simulink model "RAM_test"  (R2019a)
settings: Solver=VariableStepAuto  StartTime=0.0  StopTime=stop_time  RelTol=1e-3
InitFcn:
  | sm_callback_init
undefined symbols (not defined in the file): a, b, B_k_0_init, c, calib_bpfs, F_bits, FIR_0_Size, FIR_0_Uprate, mp, Ts, W_bits
libraries: simulink x13, dsphdlfiltering x1, hdlsllib x1
settings Model: Creator=Balad  LastModifiedBy=Bailey

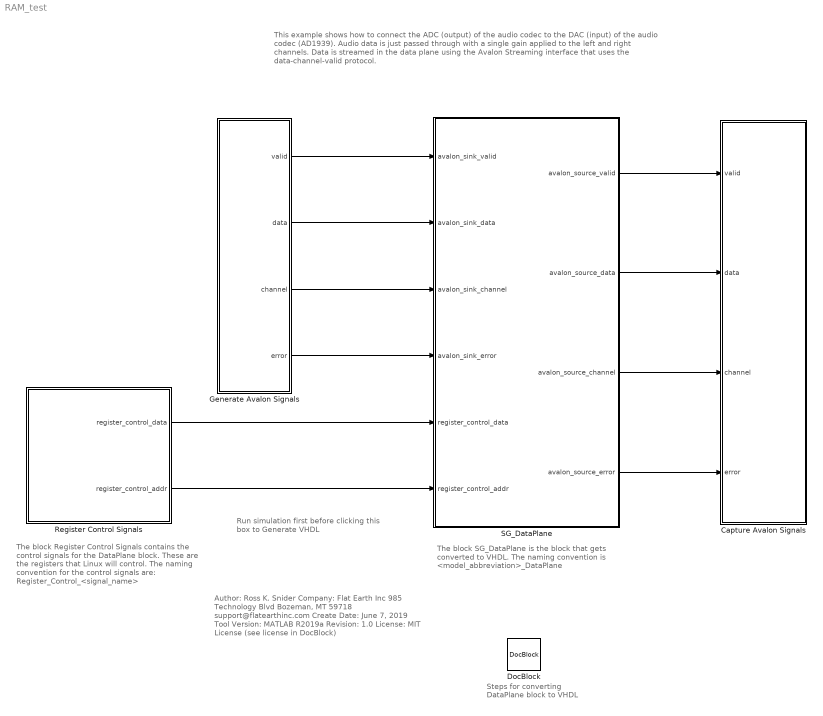
== system RAM_test ==
  note: Author:          Ross K. Snider
      | Company:     Flat Earth Inc
      |                       985 Technology Blvd
      |                       Bozeman, MT 59718
      |                       support@flatearthinc.com
      | Create Date:  June 7, 2019
      | Tool Version:  MATLAB R2019a
      | Revision:        1.0
      | License:          MIT License (see license in DocBlock)
  note: The block SG_DataPlane is the block that gets
      | converted to VHDL. The naming convention is
      | <model_abbreviation>_DataPlane
  note: Steps for converting
      | DataPlane block
      | to VHDL
  note: This example shows how to connect the ADC (output) of the audio codec to the DAC (input) of the audio codec (AD1939). Audio data is just passed through with a single gain applied to the left and right channels. Data is streamed in the data plane using the Avalon Streaming interface that uses the data-channel-valid protocol.
  note: The block Register Control Signals contains
      | the control signals for the DataPlane block.
      | These are the registers that Linux will control.
      | The naming convention for the control
      | signals are:  Register_Control_<signal_name>
  note: Run simulation first
      | before clicking this box to
      | Generate VHDL
  Capture Avalon Signals : Subsystem
  DocBlock : simulink/Model-Wide Utilities/DocBlock  DocumentType=HTML
      content=|
      | <html><head></head><body>
      | Type your documentation here</body></html>
  Generate Avalon Signals : Subsystem
  Register Control Signals : Subsystem
  SG_DataPlane : Subsystem  TreatAsAtomicUnit=on
  wires:
  Register Control Signals/2(register_control_addr) -> SG_DataPlane/6(register_control_addr)
  SG_DataPlane/2(avalon_source_data) -> Capture Avalon Signals/2(data)
  Generate Avalon Signals/3(channel) -> SG_DataPlane/3(avalon_sink_channel)
  Register Control Signals/1(register_control_data) -> SG_DataPlane/5(register_control_data)
  Generate Avalon Signals/2(data) -> SG_DataPlane/2(avalon_sink_data)
  Generate Avalon Signals/1(valid) -> SG_DataPlane/1(avalon_sink_valid)
  SG_DataPlane/4(avalon_source_error) -> Capture Avalon Signals/4(error)
  Generate Avalon Signals/4(error) -> SG_DataPlane/4(avalon_sink_error)
  SG_DataPlane/3(avalon_source_channel) -> Capture Avalon Signals/3(channel)
  SG_DataPlane/1(avalon_source_valid) -> Capture Avalon Signals/1(valid)

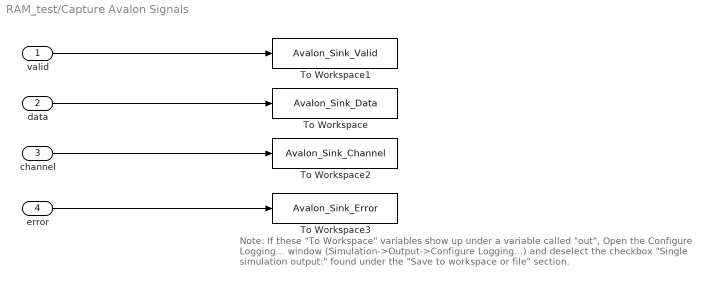
== system RAM_test/Capture Avalon Signals ==
  note: Note:  If these "To Workspace" variables show up under a variable called "out",
      | Open the Configure Logging... window (Simulation->Output->Configure Logging...)
      | and deselect the checkbox "Single simulation output:" found under the "Save to workspace or file" section.
  valid : Inport
  data : Inport  Port=2
  channel : Inport  Port=3
  error : Inport  Port=4
  To Workspace : ToWorkspace  VariableName=Avalon_Sink_Data  SaveFormat=Timeseries  SampleTime=-1
  To Workspace1 : ToWorkspace  VariableName=Avalon_Sink_Valid  SaveFormat=Timeseries  SampleTime=-1
  To Workspace2 : ToWorkspace  VariableName=Avalon_Sink_Channel  SaveFormat=Timeseries  SampleTime=-1
  To Workspace3 : ToWorkspace  VariableName=Avalon_Sink_Error  SaveFormat=Timeseries  SampleTime=-1
  wires:
  data/1 -> To Workspace/1
  valid/1 -> To Workspace1/1
  error/1 -> To Workspace3/1
  channel/1 -> To Workspace2/1

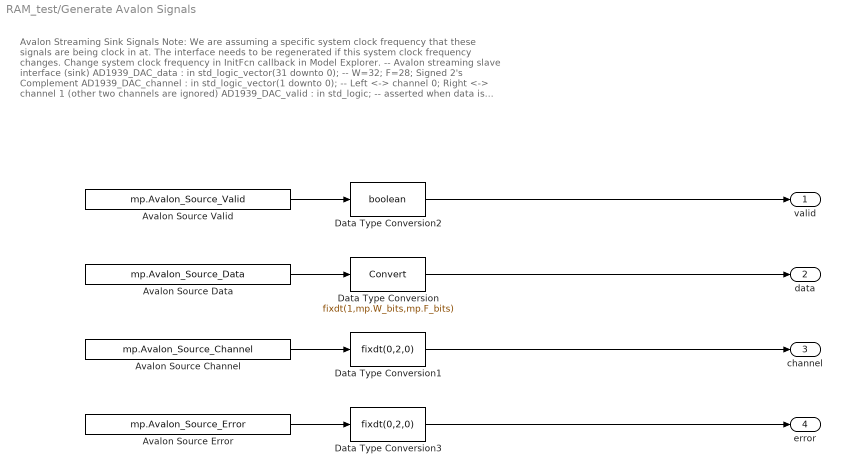
== system RAM_test/Generate Avalon Signals ==
  note: Avalon Streaming Sink Signals
      | Note: We are assuming a specific system clock frequency that these signals are being clock in at.
      | The interface needs to be regenerated if this system clock frequency changes. Change system clock frequency in InitFcn callback in Model Explorer.
      |
      | -- Avalon streaming slave interface (sink)
      | AD1939_DAC_data : in std_logic_vector(31 downto 0); -- W=32; F=28; Signed 2's Complement
      | AD1939_DAC_channel : in std_logic_vector(1 downto 0); -- Left <-> channel 0; Right <-> channel 1 (other two channels are ignored)
      | AD1939_DAC_valid : in std_logic; -- asserted when data is valid
      | AD1939_DAC_error : in std_logic_vector(1 downto 0) -- error channel is ignored, assumed to be error free at this point
      |
      | For more information on the data-channel-valid protocol, see chapter 5 in Intel's Avalon Interfaced Specification (p. 40) at https://www.intel.com/content/dam/www/programmable/us/en/pdfs/literature/manual/mnl_avalon_spec.pdf
  Avalon Source Channel : FromWorkspace  VariableName=mp.Avalon_Source_Channel  OutDataTypeStr=double  SampleTime=mp.Ts_system
  "Avalon Source Data " : FromWorkspace  VariableName=mp.Avalon_Source_Data  OutDataTypeStr=double  SampleTime=mp.Ts_system
  Avalon Source Error : FromWorkspace  VariableName=mp.Avalon_Source_Error  OutDataTypeStr=double  SampleTime=mp.Ts_system
  Avalon Source Valid : FromWorkspace  VariableName=mp.Avalon_Source_Valid  OutDataTypeStr=double  SampleTime=mp.Ts_system
  Data Type Conversion : DataTypeConversion  OutDataTypeStr=fixdt(1,mp.W_bits,mp.F_bits)
  Data Type Conversion1 : DataTypeConversion  OutDataTypeStr=fixdt(0,2,0)
  Data Type Conversion2 : DataTypeConversion  OutDataTypeStr=boolean
  Data Type Conversion3 : DataTypeConversion  OutDataTypeStr=fixdt(0,2,0)
  valid : Outport
  data : Outport  Port=2
  channel : Outport  Port=3
  error : Outport  Port=4
  wires:
  Data Type Conversion1/1 -> channel/1
  Data Type Conversion2/1 -> valid/1
  Avalon Source Error/1 -> Data Type Conversion3/1
  Data Type Conversion/1 -> data/1
  Avalon Source Valid/1 -> Data Type Conversion2/1
  Data Type Conversion3/1 -> error/1
  Avalon Source Channel/1 -> Data Type Conversion1/1
  "Avalon Source Data "/1 -> Data Type Conversion/1

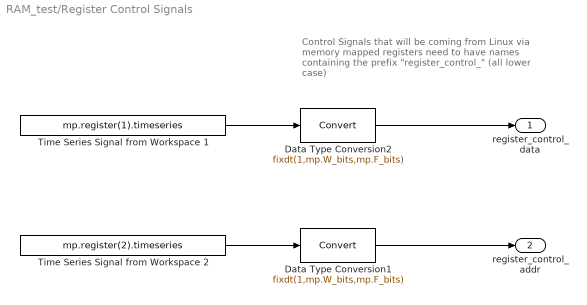
== system RAM_test/Register Control Signals ==
  note: Control Signals that will be coming from Linux via
      | memory mapped registers need to have names
      | containing the prefix "register_control_"
      | (all lower case)
  Data Type Conversion1 : DataTypeConversion  OutDataTypeStr=fixdt(1,mp.W_bits,mp.F_bits)
  Data Type Conversion2 : DataTypeConversion  OutDataTypeStr=fixdt(1,mp.W_bits,mp.F_bits)
  Time Series Signal from Workspace 1 : FromWorkspace  VariableName=mp.register(1).timeseries  OutDataTypeStr=double  SampleTime=mp.Ts_system
  Time Series Signal from Workspace 2 : FromWorkspace  VariableName=mp.register(2).timeseries  OutDataTypeStr=double  SampleTime=mp.Ts_system
  register_control_data : Outport
  register_control_addr : Outport  Port=2
  wires:
  Time Series Signal from Workspace 1/1 -> Data Type Conversion2/1
  Time Series Signal from Workspace 2/1 -> Data Type Conversion1/1
  Data Type Conversion2/1 -> register_control_data/1
  Data Type Conversion1/1 -> register_control_addr/1

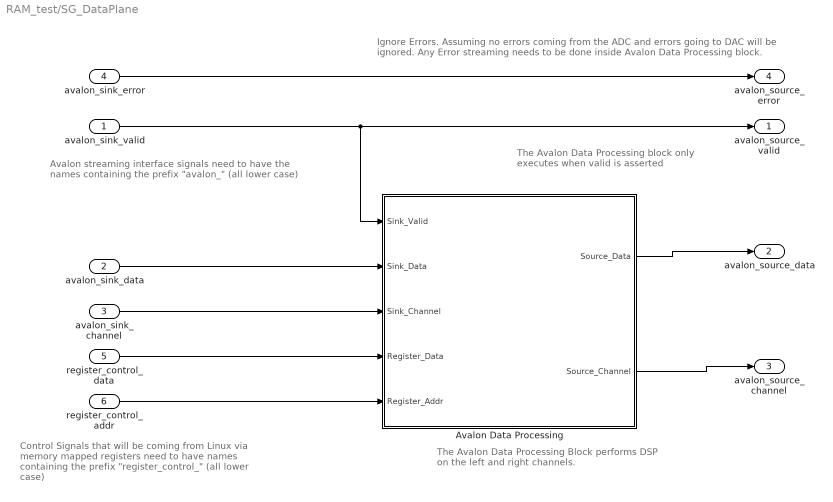
== system RAM_test/SG_DataPlane ==
  note: Control Signals that will be coming from Linux via
      | memory mapped registers need to have names
      | containing the prefix "register_control_"
      | (all lower case)
  note: The Avalon Data Processing Block
      | performs DSP on the left and right channels.
  note: The Avalon Data Processing block
      | only executes when valid is asserted
  note: Ignore Errors.
      | Assuming no errors coming from the ADC and errors going to DAC will be ignored.
      | Any Error streaming needs to be done inside Avalon Data Processing block.
  note: Avalon streaming interface signals need to have the
      | names containing the prefix "avalon_"
      | (all lower case)
  avalon_sink_valid : Inport
  avalon_sink_data : Inport  Port=2
  avalon_sink_channel : Inport  Port=3
  avalon_sink_error : Inport  Port=4
  register_control_data : Inport  Port=5
  register_control_addr : Inport  Port=6
  Avalon Data Processing : Subsystem  TreatAsAtomicUnit=on
  avalon_source_valid : Outport
  avalon_source_data : Outport  Port=2
  avalon_source_channel : Outport  Port=3
  avalon_source_error : Outport  Port=4
  wires:
  avalon_sink_channel/1 -> Avalon Data Processing/3(Sink_Channel)
  avalon_sink_error/1 -> avalon_source_error/1
  Avalon Data Processing/1(Source_Data) -> avalon_source_data/1
  avalon_sink_valid/1 -> avalon_source_valid/1, Avalon Data Processing/1(Sink_Valid)
  avalon_sink_data/1 -> Avalon Data Processing/2(Sink_Data)
  Avalon Data Processing/2(Source_Channel) -> avalon_source_channel/1
  register_control_addr/1 -> Avalon Data Processing/5(Register_Addr)
  register_control_data/1 -> Avalon Data Processing/4(Register_Data)

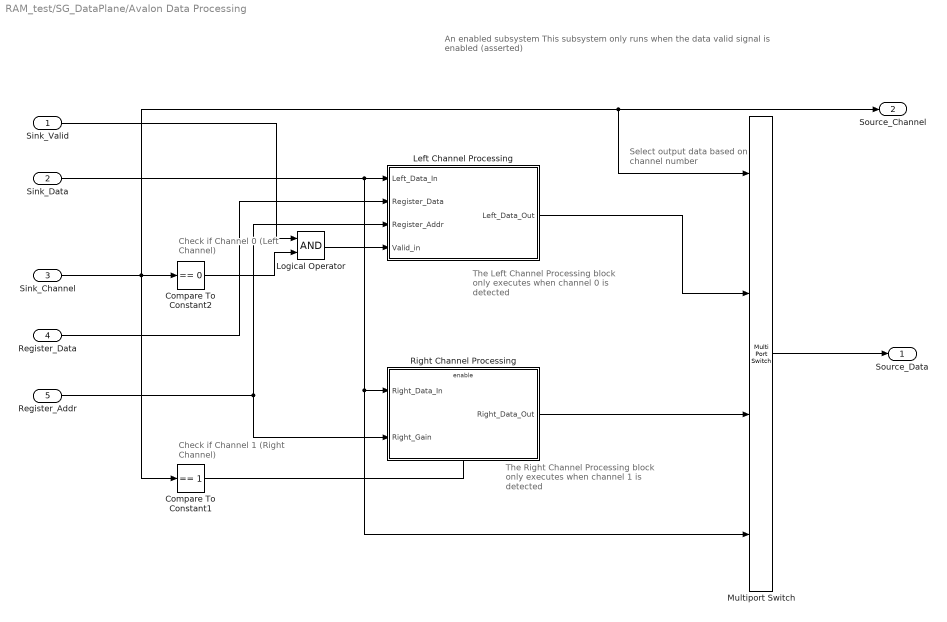
== system RAM_test/SG_DataPlane/Avalon Data Processing ==
  note: Select output data
      | based on channel number
  note: Check if Channel 0
      | (Left Channel)
  note: The Left Channel Processing block
      | only executes when channel 0
      | is detected
  note: The Right Channel Processing block
      | only executes when channel 1
      | is detected
  note: Check if Channel 1
      | (Right Channel)
  note: An enabled subsystem
      | This subsystem only runs when the data valid signal is enabled (asserted)
  Sink_Valid : Inport
  Sink_Data : Inport  Port=2
  Sink_Channel : Inport  Port=3
  Register_Data : Inport  Port=4
  Register_Addr : Inport  Port=5
  Compare To Constant1 : simulink/Logic and Bit Operations/Compare To Constant  relop===  const=1  OutDataTypeStr=boolean
  Compare To Constant2 : simulink/Logic and Bit Operations/Compare To Constant  relop===  const=0  OutDataTypeStr=boolean
  Left Channel Processing : Subsystem  TreatAsAtomicUnit=on
  Logical Operator : Logic  AllPortsSameDT=off  OutDataTypeStr=boolean
  Multiport Switch : MultiPortSwitch  DataPortOrder=Zero-based contiguous  DiagnosticForDefault=None  zeroidx=on
  Right Channel Processing : Subsystem  TreatAsAtomicUnit=on
  Source_Data : Outport  InitialOutput=0
  Source_Channel : Outport  Port=2  InitialOutput=0
  wires:
  Sink_Channel/1 -> Source_Channel/1, Multiport Switch/1, Compare To Constant1/1, Compare To Constant2/1
  Compare To Constant2/1 -> Logical Operator/2
  Compare To Constant1/1 -> Right Channel Processing/Enable
  Sink_Data/1 -> Multiport Switch/4, Right Channel Processing/1(Right_Data_In), Left Channel Processing/1(Left_Data_In)
  Left Channel Processing/1("Left_Data_Out ") -> Multiport Switch/2
  Right Channel Processing/1("Right_Data_Out ") -> Multiport Switch/3
  Multiport Switch/1 -> Source_Data/1
  Register_Data/1 -> Left Channel Processing/2(Register_Data)
  Register_Addr/1 -> Left Channel Processing/3(Register_Addr), Right Channel Processing/2(Right_Gain)
  Logical Operator/1 -> Left Channel Processing/4(Valid_in)
  Sink_Valid/1 -> Logical Operator/1

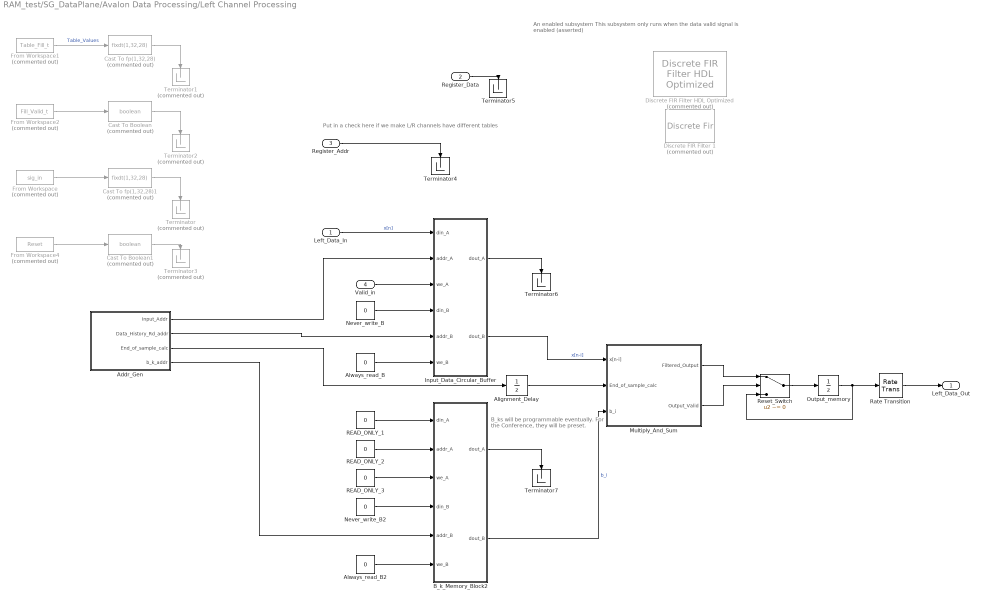
== system RAM_test/SG_DataPlane/Avalon Data Processing/Left Channel Processing ==
  note: B_ks will be programmable eventually.
      | For the Conference, they will be preset.
  note: Put in a check here if we make L/R channels have different tables
  note: An enabled subsystem
      | This subsystem only runs when the data valid signal is enabled (asserted)
  Left_Data_In : Inport
  Register_Data : Inport  Port=2
  Register_Addr : Inport  Port=3
  Valid_in : Inport  Port=4
  "Addr_Gen " : Subsystem
  Alignment_Delay : UnitDelay  SampleTime=-1  HasFrameUpgradeWarning=on
  Always_read_B : Constant  Value=0  OutDataTypeStr=boolean  SampleTime=Ts/FIR_0_Uprate
  Always_read_B2 : Constant  Value=0  OutDataTypeStr=boolean  SampleTime=Ts/FIR_0_Uprate
  B_k_Memory_Block2 : Subsystem  AncestorBlock=DualPortRam_UNLOCKED/Dual Rate Dual Port RAM1  mask(Dual-rate dual-port RAM){ram_size=FIR_0_Size}
      mask prompts: ram_size "Address port width (2 to 28 bits)"
      mask help: This block simulates a dual-clock dual-port RAM with two data output ports.
      mask init:
      | hdlblkmask_drdpram();
      mask Help: helpview([docroot '/simulink/helptargets.map'],'HDL_dual_rate_dual_port_ram');
  Cast To Boolean : DataTypeConversion  Commented=on  OutDataTypeStr=boolean
  Cast To Boolean1 : DataTypeConversion  Commented=on  OutDataTypeStr=boolean
  Cast To fp(1,32,28) : DataTypeConversion  Commented=on  OutDataTypeStr=fixdt(1,32,28)  RndMeth=Round
  Cast To fp(1,32,28)1 : DataTypeConversion  Commented=on  OutDataTypeStr=fixdt(1,32,28)  RndMeth=Round
  Discrete FIR Filter HDL Optimized : dsphdlfiltering/Discrete FIR Filter HDL Optimized  Commented=on  NumeratorSource=Property  Numerator=calib_bpfs(2:calib_bpfs(1,1)+1 ,1)'  NumeratorPrototype=[]  FilterStructure=Direct form systolic  SerializationOption=Minimum number of cycles between valid input samples  NumberOfCycles=2  NumberOfMultipliers=2  SimulateUsing=Code generation  roundingMode=Floor  overflowMode=off  CoefficientsDataTypeStr=fixdt(1, W_bits, F_bits)  CoefficientsMin=[]  CoefficientsMax=[]  OutputDataTypeStr=fixdt(1, W_bits, F_bits)  OutputMin=[]  OutputMax=[]  ResetInputPort=off  HDLGlobalReset=off
      settings: SourceProductName=DSP System Toolbox  SourceProductBaseCode=DS
  Discrete FIR Filter 1 : DiscreteFir  Commented=on  Coefficients=calib_bpfs(2:calib_bpfs(1,1)+1 ,1)'  CoefDataTypeStr=fixdt(1, W_bits, F_bits)  ProductDataTypeStr=fixdt(1, W_bits, F_bits)  AccumDataTypeStr=fixdt(1, W_bits, F_bits)  OutDataTypeStr=fixdt(1, W_bits, F_bits)
  From Workspace : FromWorkspace  Commented=on  VariableName=sig_in  SampleTime=Ts  OutputAfterFinalValue=Setting to zero
  From Workspace1 : FromWorkspace  Commented=on  VariableName=Table_Fill_t  SampleTime=Ts  Interpolate=off  OutputAfterFinalValue=Setting to zero
  From Workspace2 : FromWorkspace  Commented=on  VariableName=Fill_Valid_t  SampleTime=Ts  OutputAfterFinalValue=Setting to zero
  From Workspace4 : FromWorkspace  Commented=on  VariableName=Reset  SampleTime=Ts  Interpolate=off  OutputAfterFinalValue=Setting to zero
  Input_Data_Circular_Buffer : Subsystem  AncestorBlock=DualPortRam_UNLOCKED/Dual Rate Dual Port RAM1  mask(Dual-rate dual-port RAM){ram_size=FIR_0_Size}
      mask prompts: ram_size "Address port width (2 to 28 bits)"
      mask help: This block simulates a dual-clock dual-port RAM with two data output ports.
      mask init:
      | hdlblkmask_drdpram();
      mask Help: helpview([docroot '/simulink/helptargets.map'],'HDL_dual_rate_dual_port_ram');
  Multiply_And_Sum : Subsystem
  Never_write_B : Constant  Value=0  OutDataTypeStr=fixdt(1,W_bits, F_bits)  SampleTime=Ts/FIR_0_Uprate
  Never_write_B2 : Constant  Value=0  OutDataTypeStr=fixdt(1,W_bits, F_bits)  SampleTime=Ts/FIR_0_Uprate
  Output_memory : UnitDelay  SampleTime=-1  HasFrameUpgradeWarning=on
  READ_ONLY_1 : Constant  Value=0  OutDataTypeStr=fixdt(1,W_bits, F_bits)  SampleTime=Ts/FIR_0_Uprate
  READ_ONLY_2 : Constant  Value=0  OutDataTypeStr=fixdt(0,FIR_0_Size, 0)  SampleTime=Ts/FIR_0_Uprate
  READ_ONLY_3 : Constant  Value=0  OutDataTypeStr=boolean  SampleTime=Ts/FIR_0_Uprate
  Rate Transition : RateTransition  OutPortSampleTime=Ts
  Reset_Switch : Switch  Criteria=u2 ~= 0
  Terminator{,1..3} (4 alike) : Terminator  Commented=on
  Terminator{4..7} (4 alike) : Terminator
  "Left_Data_Out " : Outport  InitialOutput=0
  wires:
  Cast To Boolean1/1 -> Terminator3/1
  Cast To Boolean/1 -> Terminator2/1
  Cast To fp(1,32,28)1/1 -> Terminator/1
  From Workspace1/1 -> Cast To fp(1,32,28)/1  "Table_Values"
  Output_memory/1 -> Rate Transition/1, Reset_Switch/3
  From Workspace2/1 -> Cast To Boolean/1
  From Workspace/1 -> Cast To fp(1,32,28)1/1
  From Workspace4/1 -> Cast To Boolean1/1
  Cast To fp(1,32,28)/1 -> Terminator1/1
  Left_Data_In/1 -> Input_Data_Circular_Buffer/1(din_A)  "x[n]"
  Register_Data/1 -> Terminator5/1
  Register_Addr/1 -> Terminator4/1
  Valid_in/1 -> Input_Data_Circular_Buffer/3(we_A)
  Input_Data_Circular_Buffer/1(dout_A) -> Terminator6/1
  Never_write_B/1 -> Input_Data_Circular_Buffer/4(din_B)
  "Addr_Gen "/1(Input_Addr) -> Input_Data_Circular_Buffer/2(addr_A)
  "Addr_Gen "/2(Data_History_Rd_addr) -> Input_Data_Circular_Buffer/5(addr_B)
  Always_read_B/1 -> Input_Data_Circular_Buffer/6(we_B)
  Input_Data_Circular_Buffer/2(dout_B) -> Multiply_And_Sum/1(x[n-i])  "x[n-i]"
  READ_ONLY_1/1 -> B_k_Memory_Block2/1(din_A)
  READ_ONLY_3/1 -> B_k_Memory_Block2/3(we_A)
  READ_ONLY_2/1 -> B_k_Memory_Block2/2(addr_A)
  Never_write_B2/1 -> B_k_Memory_Block2/4(din_B)
  "Addr_Gen "/4(b_k_addr) -> B_k_Memory_Block2/5(addr_B)
  Always_read_B2/1 -> B_k_Memory_Block2/6(we_B)
  B_k_Memory_Block2/1(dout_A) -> Terminator7/1
  B_k_Memory_Block2/2(dout_B) -> Multiply_And_Sum/3(b_i)  "b_i"
  "Addr_Gen "/3(End_of_sample_calc) -> Alignment_Delay/1
  Reset_Switch/1 -> Output_memory/1
  Multiply_And_Sum/2(Output_Valid) -> Reset_Switch/2
  Multiply_And_Sum/1(Filtered_Output) -> Reset_Switch/1
  Rate Transition/1 -> "Left_Data_Out "/1
  Alignment_Delay/1 -> Multiply_And_Sum/2(End_of_sample_calc)

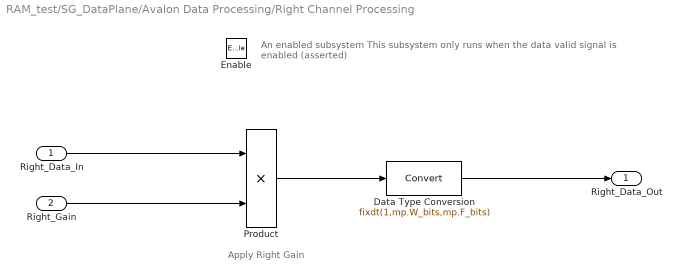
== system RAM_test/SG_DataPlane/Avalon Data Processing/Right Channel Processing ==
  note: Apply Right Gain
  note: An enabled subsystem
      | This subsystem only runs when the data valid signal is enabled (asserted)
  Right_Data_In : Inport
  Right_Gain : Inport  Port=2
  Enable : EnablePort
  Data Type Conversion : DataTypeConversion  OutDataTypeStr=fixdt(1,mp.W_bits,mp.F_bits)
  Product : Product
  "Right_Data_Out " : Outport  InitialOutput=0
  wires:
  Data Type Conversion/1 -> "Right_Data_Out "/1
  Product/1 -> Data Type Conversion/1
  Right_Data_In/1 -> Product/1
  Right_Gain/1 -> Product/2

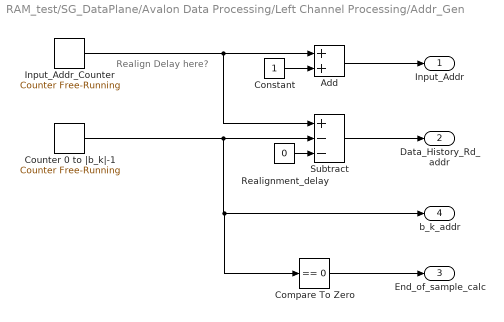
== system RAM_test/SG_DataPlane/Avalon Data Processing/Left Channel Processing/Addr_Gen  ==
  note: Realign Delay here?
  Add : Sum  OutDataTypeStr=Inherit: Same as first input
  Compare To Zero : simulink/Logic and Bit Operations/Compare To Zero  relop===  OutDataTypeStr=boolean  ZeroCross=off
  Constant : Constant  OutDataTypeStr=fixdt(0, FIR_0_Size,0)  SampleTime=-1
  Counter 0 to |b_k|-1 : simulink/Sources/Counter Free-Running  NumBits=FIR_0_Size  tsamp=Ts/FIR_0_Uprate
  Input_Addr_Counter : simulink/Sources/Counter Free-Running  NumBits=FIR_0_Size  tsamp=Ts
  Realignment_delay : Constant  Value=0  OutDataTypeStr=fixdt(0, FIR_0_Size,0)  SampleTime=-1
  Subtract : Sum  Inputs=+--  OutDataTypeStr=Inherit: Same as first input
  Input_Addr : Outport
  Data_History_Rd_addr : Outport  Port=2
  End_of_sample_calc : Outport  Port=3
  b_k_addr : Outport  Port=4
  wires:
  Counter 0 to |b_k|-1/1 -> Subtract/2, Compare To Zero/1, b_k_addr/1
  Subtract/1 -> Data_History_Rd_addr/1
  Input_Addr_Counter/1 -> Add/1, Subtract/1
  Add/1 -> Input_Addr/1
  Constant/1 -> Add/2
  Realignment_delay/1 -> Subtract/3
  Compare To Zero/1 -> End_of_sample_calc/1

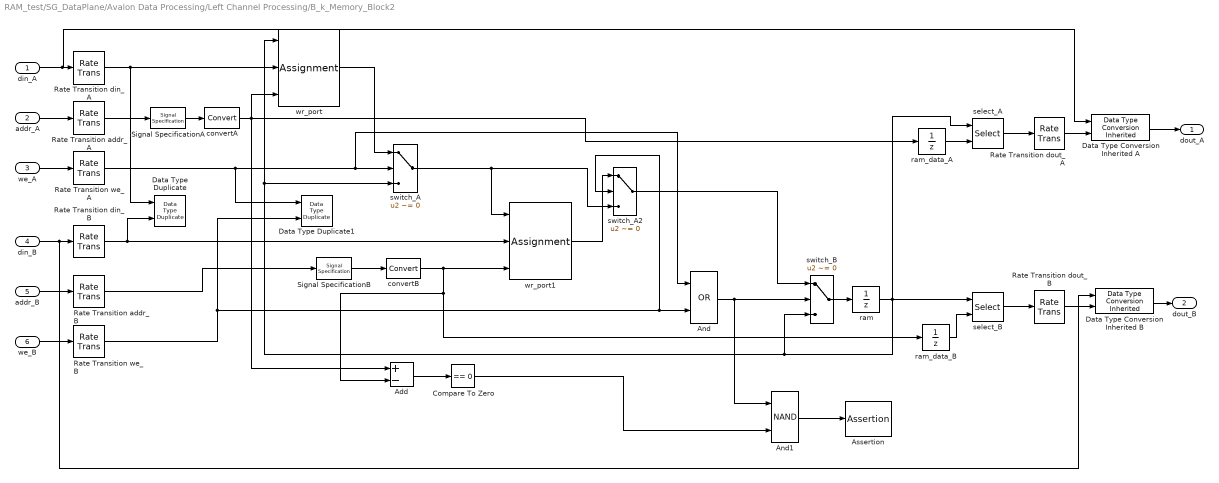
== system RAM_test/SG_DataPlane/Avalon Data Processing/Left Channel Processing/B_k_Memory_Block2 ==
  din_A : Inport
  addr_A : Inport  Port=2
  we_A : Inport  Port=3  OutDataTypeStr=boolean
  din_B : Inport  Port=4
  addr_B : Inport  Port=5
  we_B : Inport  Port=6  OutDataTypeStr=boolean
  Add : Sum  Inputs=+-
  And : Logic  Operator=OR  AllPortsSameDT=off  OutDataTypeStr=boolean
  And1 : Logic  Operator=NAND  AllPortsSameDT=off  OutDataTypeStr=boolean
  Assertion : Assertion  StopWhenAssertionFail=off
  Compare To Zero : simulink/Logic and Bit Operations/Compare To Zero  relop===  OutDataTypeStr=boolean
  Data Type Conversion Inherited A : simulink/Signal Attributes/Data Type Conversion Inherited  ConvertRealWorld=Real World Value  DoSatur=off
      settings: SourceProductName=Simulink  SourceProductBaseCode=SL
  Data Type Conversion Inherited B : simulink/Signal Attributes/Data Type Conversion Inherited  ConvertRealWorld=Real World Value  DoSatur=off
      settings: SourceProductName=Simulink  SourceProductBaseCode=SL
  Data Type Duplicate : DataTypeDuplicate
  Data Type Duplicate1 : DataTypeDuplicate
  Rate Transition addr_A : RateTransition  Integrity=off
  Rate Transition addr_B : RateTransition  Integrity=off
  Rate Transition din_A : RateTransition  Integrity=off
  Rate Transition din_B : RateTransition  Integrity=off
  Rate Transition dout_A : RateTransition  Integrity=off
  Rate Transition dout_B : RateTransition  Integrity=off
  Rate Transition we_A : RateTransition  Integrity=off
  Rate Transition we_B : RateTransition  Integrity=off
  Signal SpecificationA : SignalSpecification  OutDataTypeStr=fixdt(0,ram_size,0)  Dimensions=1
  Signal SpecificationB : SignalSpecification  OutDataTypeStr=fixdt(0,ram_size,0)  Dimensions=1
  convertA : DataTypeConversion
  convertB : DataTypeConversion
  ram : UnitDelay  InitialCondition=B_k_0_init  SampleTime=-1  HasFrameUpgradeWarning=on
  ram_data_A : UnitDelay  SampleTime=-1  HasFrameUpgradeWarning=on
  ram_data_B : UnitDelay  SampleTime=-1  HasFrameUpgradeWarning=on
  select_A : Selector  IndexMode=Zero-based  InputPortWidth=2^ram_size  IndexOptions=Index vector (port)  Indices=[1 3]  OutputSizes=1
  select_B : Selector  IndexMode=Zero-based  InputPortWidth=2^ram_size  IndexOptions=Index vector (port)  Indices=[1 3]  OutputSizes=1
  switch_A : Switch  Criteria=u2 ~= 0
  switch_A2 : Switch  Criteria=u2 ~= 0
  switch_B : Switch  Criteria=u2 ~= 0
  wr_port : Assignment  IndexMode=Zero-based  IndexOptions=Index vector (port)  Indices=1  OutputSizes=[1 1]
  wr_port1 : Assignment  IndexMode=Zero-based  IndexOptions=Index vector (port)  Indices=1  OutputSizes=[1 1]
  dout_A : Outport
  dout_B : Outport  Port=2
  wires:
  we_A/1 -> Rate Transition we_A/1
  select_A/1 -> Rate Transition dout_A/1
  switch_A2/1 -> switch_B/1
  And1/1 -> Assertion/1
  Signal SpecificationA/1 -> convertA/1
  Signal SpecificationB/1 -> convertB/1
  din_B/1 -> Data Type Conversion Inherited B/1, Rate Transition din_B/1
  switch_B/1 -> ram/1
  addr_B/1 -> Rate Transition addr_B/1
  convertA/1 -> ram_data_A/1, wr_port/3, Add/1
  we_B/1 -> Rate Transition we_B/1
  ram/1 -> select_B/1, switch_B/3, switch_A/3, wr_port/1, select_A/1
  wr_port/1 -> switch_A/1
  And/1 -> And1/1, switch_B/2
  wr_port1/1 -> switch_A2/1
  Add/1 -> Compare To Zero/1
  Compare To Zero/1 -> And1/2
  Rate Transition we_B/1 -> switch_A2/2, And/2, Data Type Duplicate1/2
  switch_A/1 -> wr_port1/1, switch_A2/3
  Rate Transition addr_B/1 -> Signal SpecificationB/1
  select_B/1 -> Rate Transition dout_B/1
  ram_data_B/1 -> select_B/2
  Rate Transition we_A/1 -> Data Type Duplicate1/1, And/1, switch_A/2
  ram_data_A/1 -> select_A/2
  Rate Transition din_A/1 -> Data Type Duplicate/1, wr_port/2
  convertB/1 -> ram_data_B/1, Add/2, wr_port1/3
  din_A/1 -> Data Type Conversion Inherited A/1, Rate Transition din_A/1
  Rate Transition din_B/1 -> wr_port1/2, Data Type Duplicate/2
  addr_A/1 -> Rate Transition addr_A/1
  Rate Transition addr_A/1 -> Signal SpecificationA/1
  Rate Transition dout_B/1 -> Data Type Conversion Inherited B/2
  Data Type Conversion Inherited B/1 -> dout_B/1
  Rate Transition dout_A/1 -> Data Type Conversion Inherited A/2
  Data Type Conversion Inherited A/1 -> dout_A/1

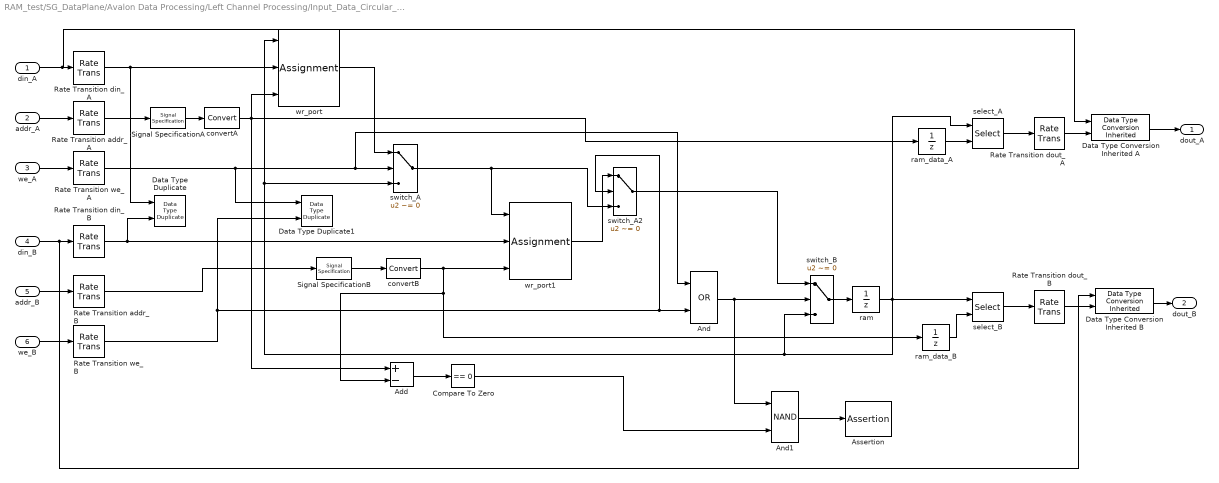
== system RAM_test/SG_DataPlane/Avalon Data Processing/Left Channel Processing/Input_Data_Circular_Buffer ==
  din_A : Inport
  addr_A : Inport  Port=2
  we_A : Inport  Port=3  OutDataTypeStr=boolean
  din_B : Inport  Port=4
  addr_B : Inport  Port=5
  we_B : Inport  Port=6  OutDataTypeStr=boolean
  Add : Sum  Inputs=+-
  And : Logic  Operator=OR  AllPortsSameDT=off  OutDataTypeStr=boolean
  And1 : Logic  Operator=NAND  AllPortsSameDT=off  OutDataTypeStr=boolean
  Assertion : Assertion  StopWhenAssertionFail=off
  Compare To Zero : simulink/Logic and Bit Operations/Compare To Zero  relop===  OutDataTypeStr=boolean
  Data Type Conversion Inherited A : simulink/Signal Attributes/Data Type Conversion Inherited  ConvertRealWorld=Real World Value  DoSatur=off
      settings: SourceProductName=Simulink  SourceProductBaseCode=SL
  Data Type Conversion Inherited B : simulink/Signal Attributes/Data Type Conversion Inherited  ConvertRealWorld=Real World Value  DoSatur=off
      settings: SourceProductName=Simulink  SourceProductBaseCode=SL
  Data Type Duplicate : DataTypeDuplicate
  Data Type Duplicate1 : DataTypeDuplicate
  Rate Transition addr_A : RateTransition  Integrity=off
  Rate Transition addr_B : RateTransition  Integrity=off
  Rate Transition din_A : RateTransition  Integrity=off
  Rate Transition din_B : RateTransition  Integrity=off
  Rate Transition dout_A : RateTransition  Integrity=off
  Rate Transition dout_B : RateTransition  Integrity=off
  Rate Transition we_A : RateTransition  Integrity=off
  Rate Transition we_B : RateTransition  Integrity=off
  Signal SpecificationA : SignalSpecification  OutDataTypeStr=fixdt(0,ram_size,0)  Dimensions=1
  Signal SpecificationB : SignalSpecification  OutDataTypeStr=fixdt(0,ram_size,0)  Dimensions=1
  convertA : DataTypeConversion
  convertB : DataTypeConversion
  ram : UnitDelay  SampleTime=-1  HasFrameUpgradeWarning=on
  ram_data_A : UnitDelay  SampleTime=-1  HasFrameUpgradeWarning=on
  ram_data_B : UnitDelay  SampleTime=-1  HasFrameUpgradeWarning=on
  select_A : Selector  IndexMode=Zero-based  InputPortWidth=2^ram_size  IndexOptions=Index vector (port)  Indices=[1 3]  OutputSizes=1
  select_B : Selector  IndexMode=Zero-based  InputPortWidth=2^ram_size  IndexOptions=Index vector (port)  Indices=[1 3]  OutputSizes=1
  switch_A : Switch  Criteria=u2 ~= 0
  switch_A2 : Switch  Criteria=u2 ~= 0
  switch_B : Switch  Criteria=u2 ~= 0
  wr_port : Assignment  IndexMode=Zero-based  IndexOptions=Index vector (port)  Indices=1  OutputSizes=[1 1]
  wr_port1 : Assignment  IndexMode=Zero-based  IndexOptions=Index vector (port)  Indices=1  OutputSizes=[1 1]
  dout_A : Outport
  dout_B : Outport  Port=2
  wires:
  Data Type Conversion Inherited A/1 -> dout_A/1
  Rate Transition dout_A/1 -> Data Type Conversion Inherited A/2
  Data Type Conversion Inherited B/1 -> dout_B/1
  Rate Transition dout_B/1 -> Data Type Conversion Inherited B/2
  Rate Transition addr_A/1 -> Signal SpecificationA/1
  addr_A/1 -> Rate Transition addr_A/1
  Rate Transition din_B/1 -> Data Type Duplicate/2, wr_port1/2
  din_A/1 -> Rate Transition din_A/1, Data Type Conversion Inherited A/1
  convertB/1 -> wr_port1/3, Add/2, ram_data_B/1
  Rate Transition din_A/1 -> wr_port/2, Data Type Duplicate/1
  ram_data_A/1 -> select_A/2
  Rate Transition we_A/1 -> switch_A/2, And/1, Data Type Duplicate1/1
  ram_data_B/1 -> select_B/2
  select_B/1 -> Rate Transition dout_B/1
  Rate Transition addr_B/1 -> Signal SpecificationB/1
  switch_A/1 -> switch_A2/3, wr_port1/1
  Rate Transition we_B/1 -> Data Type Duplicate1/2, And/2, switch_A2/2
  Compare To Zero/1 -> And1/2
  Add/1 -> Compare To Zero/1
  wr_port1/1 -> switch_A2/1
  And/1 -> switch_B/2, And1/1
  wr_port/1 -> switch_A/1
  ram/1 -> select_A/1, wr_port/1, switch_A/3, switch_B/3, select_B/1
  we_B/1 -> Rate Transition we_B/1
  convertA/1 -> Add/1, wr_port/3, ram_data_A/1
  addr_B/1 -> Rate Transition addr_B/1
  switch_B/1 -> ram/1
  din_B/1 -> Rate Transition din_B/1, Data Type Conversion Inherited B/1
  Signal SpecificationB/1 -> convertB/1
  Signal SpecificationA/1 -> convertA/1
  And1/1 -> Assertion/1
  switch_A2/1 -> switch_B/1
  select_A/1 -> Rate Transition dout_A/1
  we_A/1 -> Rate Transition we_A/1

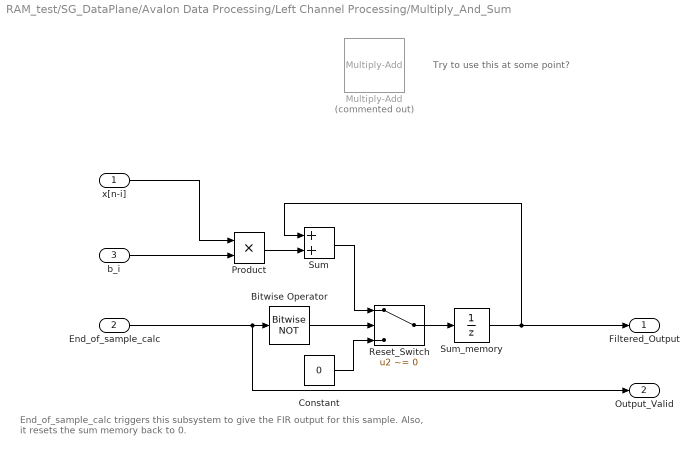
== system RAM_test/SG_DataPlane/Avalon Data Processing/Left Channel Processing/Multiply_And_Sum ==
  note: Try to use this at some point?
  note: End_of_sample_calc triggers this subsystem to give the FIR output for this sample.
      | Also, it resets the sum memory back to 0.
  x[n-i] : Inport
  End_of_sample_calc : Inport  Port=2
  b_i : Inport  Port=3
  Bitwise Operator : simulink/Logic and Bit Operations/Bitwise Operator  logicop=NOT  UseBitMask=off  BitMaskRealWorld=Stored Integer
  Constant : Constant  Value=0  OutDataTypeStr=fixdt(1, W_bits, F_bits)  SampleTime=Ts/FIR_0_Uprate
  Multiply-Add : hdlsllib/HDL Operations/Multiply-Add  Commented=on  Function=c+(a.*b)  datatype=Inherit: Inherit via internal rule  DoSatur=off  FMA=off
      settings: SourceProductName=Simulink  SourceProductBaseCode=SL
  Product : Product
  Reset_Switch : Switch  Criteria=u2 ~= 0  ZeroCross=off
  Sum : Sum  OutDataTypeStr=Inherit: Same as first input
  Sum_memory : UnitDelay  SampleTime=-1  HasFrameUpgradeWarning=on
  Filtered_Output : Outport
  Output_Valid : Outport  Port=2
  wires:
  x[n-i]/1 -> Product/1
  End_of_sample_calc/1 -> Output_Valid/1, Bitwise Operator/1
  b_i/1 -> Product/2
  Product/1 -> Sum/2
  Sum_memory/1 -> Filtered_Output/1, Sum/1
  Sum/1 -> Reset_Switch/1
  Reset_Switch/1 -> Sum_memory/1
  Constant/1 -> Reset_Switch/3
  Bitwise Operator/1 -> Reset_Switch/2
